simulink model "stringStabilityTestCreator"  (R2018b)
settings: Solver=VariableStepAuto  StartTime=0.0  StopTime=240  RelTol=1e-3
settings Model: Creator=ckreienk  LastModifiedBy=ckreienk

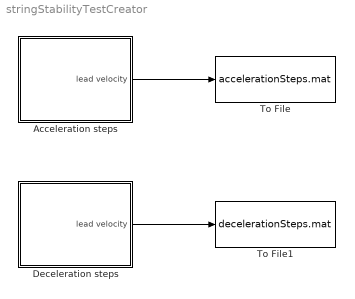
== system stringStabilityTestCreator ==
  Acceleration steps : Subsystem
  Deceleration steps : Subsystem
  To File : ToFile  Filename=accelerationSteps.mat  SaveFormat=Timeseries
  To File1 : ToFile  Filename=decelerationSteps.mat  SaveFormat=Timeseries
  wires:
  Acceleration steps/1(lead velocity) -> To File/1
  Deceleration steps/1(lead velocity) -> To File1/1

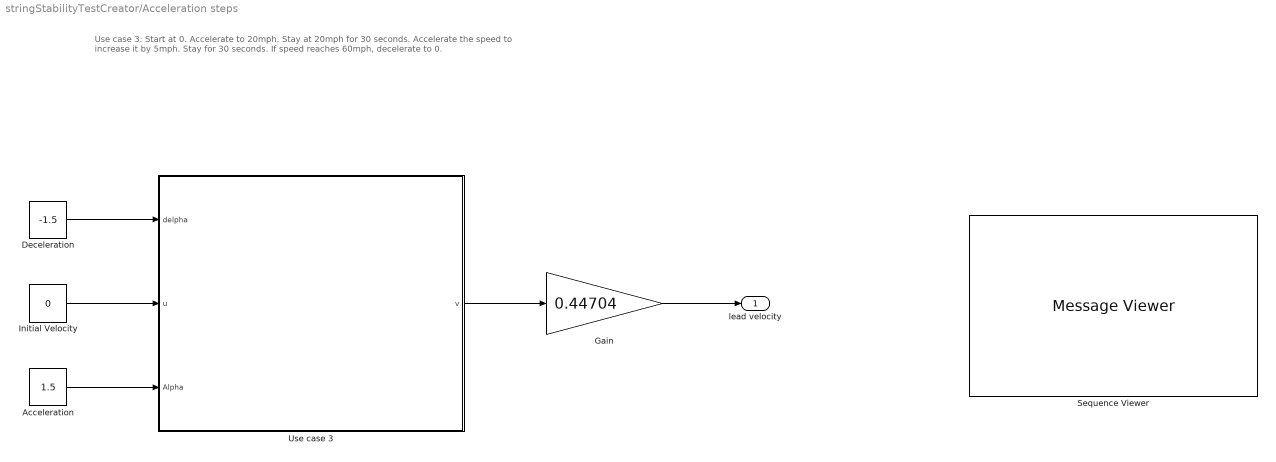
== system stringStabilityTestCreator/Acceleration steps ==
  note: Use case 3:
      | Start at 0. Accelerate to 20mph. Stay at 20mph for 30 seconds.
      | Accelerate the speed to increase it by 5mph. Stay for 30 seconds.
      | If speed reaches 60mph, decelerate to 0.
  Acceleration : Constant  Value=1.5
  Deceleration : Constant  Value=-1.5
  Gain : Gain  Gain=0.44704
  Initial Velocity : Constant  Value=0
  Sequence Viewer : MessageViewer
  Use case 3 : Stateflow chart  TreatAsAtomicUnit=on
  lead velocity : Outport
  wires:
  Acceleration/1 -> Use case 3/3(Alpha)
  Initial Velocity/1 -> Use case 3/2(u)
  Deceleration/1 -> Use case 3/1(delpha)
  Use case 3/1(v) -> Gain/1
  Gain/1 -> lead velocity/1

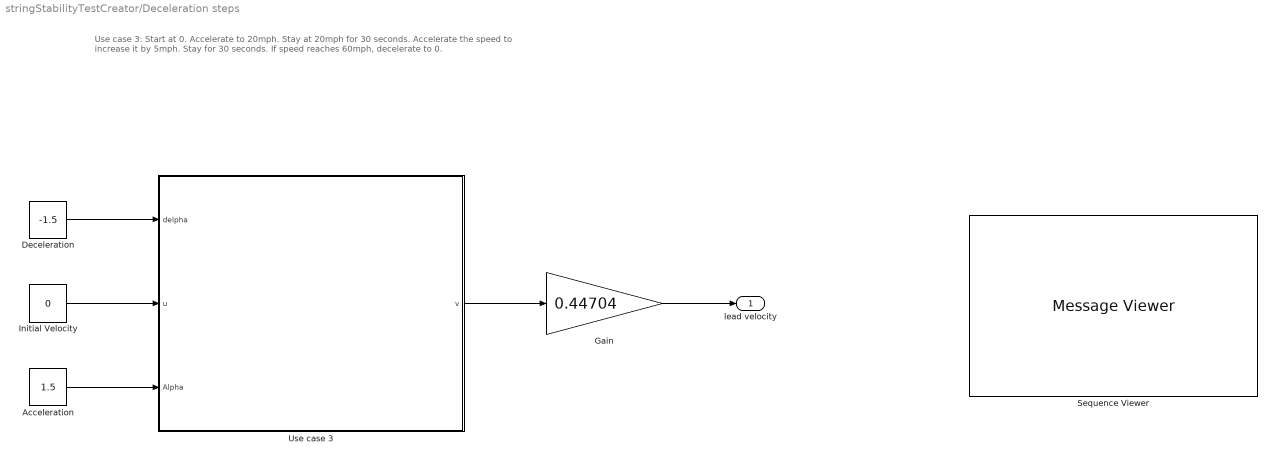
== system stringStabilityTestCreator/Deceleration steps ==
  note: Use case 3:
      | Start at 0. Accelerate to 20mph. Stay at 20mph for 30 seconds.
      | Accelerate the speed to increase it by 5mph. Stay for 30 seconds.
      | If speed reaches 60mph, decelerate to 0.
  Acceleration : Constant  Value=1.5
  Deceleration : Constant  Value=-1.5
  Gain : Gain  Gain=0.44704
  Initial Velocity : Constant  Value=0
  Sequence Viewer : MessageViewer
  Use case 3 : Stateflow chart  TreatAsAtomicUnit=on
  lead velocity : Outport
  wires:
  Use case 3/1(v) -> Gain/1
  Deceleration/1 -> Use case 3/1(delpha)
  Initial Velocity/1 -> Use case 3/2(u)
  Acceleration/1 -> Use case 3/3(Alpha)
  Gain/1 -> lead velocity/1

== stateflow chart stringStabilityTestCreator/Acceleration steps/Use case 3 ==
  note: Use case 3:
      | Start at 0. Accelerate to 20mph. Stay at 20mph for 30 seconds.
      | Accelerate the speed to increase it by 5mph. Stay for 30 seconds.
      | If speed reaches 60mph, decelerate to 0.
  state DecelerateTo0
    entry: entryState = nextState;
    during: v = getNewVaccel(v, delpha);
    exit: nextState = entryState + 1;
    note: STATE 3
  state zero
    entry: v = 0;
    during:v = 0;
    note: STATE 4
  state Accelerate
    entry: entryState = nextState; v = u2;
    during: v = getNewVaccel(v, Alpha);
    exit: nextState = entryState + 1;
    note: STATE 2
  state AccelerateTo60_init
    entry: entryState = 1; v = u;
    during: v = getNewVaccel(v, Alpha)
    exit:  nextState = entryState + 1;
    note: STATE 1
  state Hold
    entry: u2 = v;
    during: v = u2;
    exit:
    note: HOLD STATE
  DecelerateTo0 -> zero : [v <=0]
  Accelerate -> DecelerateTo0 [order 2] : [v > 35]
  Accelerate -> Hold [order 1] : [v - u2 >= 5 && v <= 35 ]
  Hold -> Accelerate : [after(30, sec)]
  (default) -> AccelerateTo60_init
  AccelerateTo60_init -> Hold : [v>=5 ]
  data: init_velocity function_input; acceleration function_input; new_vel function_output; delpha input; u input; Alpha input; v output =0; u2 local =0; entryState local =0; nextState local =0
  function new_vel = getNewVaccel(init_velocity, acceleration):
    | function new_vel = getNewVaccel(init_velocity, acceleration)
    | 
    | new_vel = init_velocity + (acceleration*0.05);
    | 
    | end

== stateflow chart stringStabilityTestCreator/Deceleration steps/Use case 3 ==
  note: Use case 3:
      | Start at 0. Accelerate to 20mph. Stay at 20mph for 30 seconds.
      | Accelerate the speed to increase it by 5mph. Stay for 30 seconds.
      | If speed reaches 60mph, decelerate to 0.
  state DecelerateTo0
    entry: entryState = nextState;
    during: v = getNewVdecel(v, delpha);
    exit: nextState = entryState + 1;
    note: STATE 3
  state zero
    entry: v = 0;
    during:v = 0;
    note: STATE 4
  state Accelerate
    entry: entryState = nextState; v = u2;
    during: v = getNewVdecel(v, Alpha);
    exit: nextState = entryState + 1;
    note: STATE 2
  state AccelerateTo60_init
    entry: entryState = 1; v = u;
    during: v = getNewVaccel(v, Alpha)
    exit:  nextState = entryState + 1;
    note: STATE 1
  state Hold
    entry: u2 = v;
    during: v = u2;
    exit:
    note: HOLD STATE
  DecelerateTo0 -> zero : [v <=0]
  Accelerate -> DecelerateTo0 [order 2] : [v < 5]
  Accelerate -> Hold [order 1] : [u2 - v >= 5 && v >= 5 ]
  Hold -> Accelerate : [after(30, sec)]
  (default) -> AccelerateTo60_init
  AccelerateTo60_init -> Hold : [v>=35 ]
  data: init_velocity function_input; deceleration function_input; new_vel function_output; init_velocity function_input; acceleration function_input; new_vel function_output; delpha input; u input; Alpha input; v output =0; u2 local =0; entryState local =0; nextState local =0
  function new_vel = getNewVdecel(init_velocity, deceleration):
    | function new_vel = getNewVdecel(init_velocity, deceleration)
    | 
    | new_vel = init_velocity - abs(deceleration*0.05);
    | 
    | end
  function new_vel = getNewVaccel(init_velocity, acceleration):
    | function new_vel = getNewVaccel(init_velocity, acceleration)
    | 
    | new_vel = init_velocity + (acceleration*0.05);
    | 
    | end
